simulink model "dynamik_6DoF"  (R2025b)
settings: Solver=VariableStepAuto  StartTime=0.0  StopTime=10.0  RelTol=1e-3
undefined symbols (not defined in the file): g, h0, Ivec, m
settings Model: Creator=chris  LastModifiedBy=chris
settings ModelReferenceCC: ModelReferenceMinAlgLoopOccurrences=on

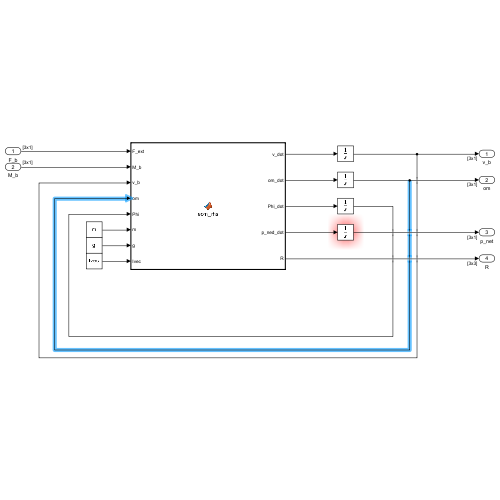
[thumbnail: Simulink's stored preview of the top-level diagram]
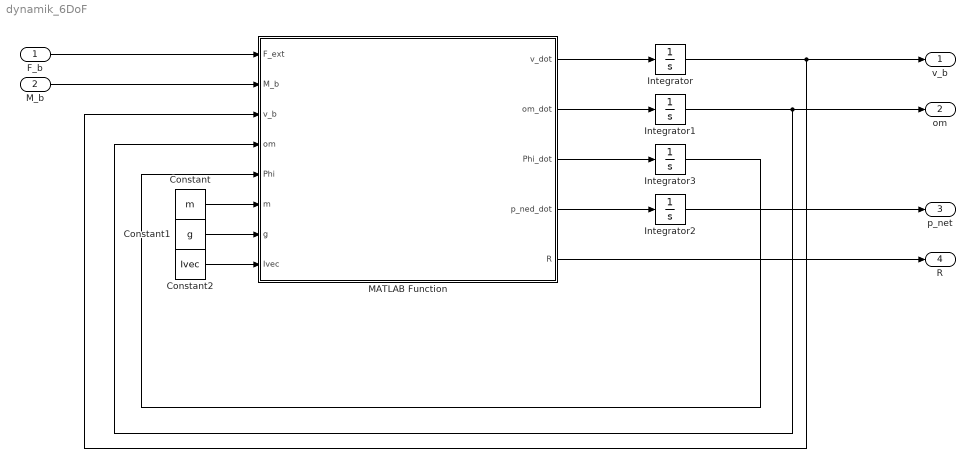
== system dynamik_6DoF ==
  F_b : Inport  PortDimensions=[3 1]
  M_b : Inport  Port=2  PortDimensions=[3 1]
  Constant : Constant  Value=m
  Constant1 : Constant  Value=g
  Constant2 : Constant  Value=Ivec
  Integrator : Integrator  InitialCondition=[0;0;0]
  Integrator1 : Integrator  InitialCondition=[0;0;0]
  Integrator2 : Integrator  InitialCondition=[0;0;-h0]
  Integrator3 : Integrator  InitialCondition=[0;0;0]
  MATLAB Function : MATLAB Function  TreatAsAtomicUnit=on
  v_b : Outport  PortDimensions=[3 1]
  om : Outport  Port=2  PortDimensions=[3 1]
  p_net : Outport  Port=3  PortDimensions=[3 1]
  R : Outport  Port=4  PortDimensions=[3 3]
  wires:
  F_b/1 -> MATLAB Function/1(F_ext)
  M_b/1 -> MATLAB Function/2(M_b)
  MATLAB Function/1(v_dot) -> Integrator/1
  MATLAB Function/2(om_dot) -> Integrator1/1
  MATLAB Function/4(p_ned_dot) -> Integrator2/1
  MATLAB Function/3(Phi_dot) -> Integrator3/1
  Integrator/1 -> v_b/1, MATLAB Function/3(v_b)
  Integrator1/1 -> om/1, MATLAB Function/4(om)
  Integrator3/1 -> MATLAB Function/5(Phi)
  Constant/1 -> MATLAB Function/6(m)
  Constant1/1 -> MATLAB Function/7(g)
  Constant2/1 -> MATLAB Function/8(Ivec)
  MATLAB Function/5(R) -> R/1
  Integrator2/1 -> p_net/1

== matlab function dynamik_6DoF/MATLAB Function ==
  data: F_ext input; v_dot output; M_b input; v_b input; om input; Phi input; m input; g input; Ivec input; om_dot output; Phi_dot output size=[3 1]; p_ned_dot output; R output
function [v_dot, om_dot, Phi_dot, p_ned_dot, R] = eom_rhs(F_ext, M_b, v_b, om, Phi, m, g, Ivec)
% Rechte Seite aller 12 DGL. F_ext = Schub + Drag (Body), OHNE Gravitation.
phi = Phi(1); the = Phi(2); psi = Phi(3);
cph=cos(phi); sph=sin(phi); cth=cos(the); sth=sin(the); cps=cos(psi); sps=sin(psi);

% Rotationsmatrix Body->NED (ZYX), Gl. (4.5)
R = [cth*cps, sph*sth*cps-cph*sps, cph*sth*cps+sph*sps;
     cth*sps, sph*sth*sps+cph*cps, cph*sth*sps-sph*cps;
    -sth,     sph*cth,             cph*cth];

% Gravitation in den Body-Frame drehen (R' = NED->Body)
F_grav_b = R.' * [0; 0; m*g];

v_dot     = (F_ext + F_grav_b)/m - cross(om, v_b);   % (4.1)
om_dot    = (M_b - cross(om, Ivec.*om)) ./ Ivec;     % (4.2)
W = [1, sph*tan(the), cph*tan(the);                  % (4.3) Sing. bei the=±pi/2
     0, cph,         -sph;
     0, sph/cth,      cph/cth];
Phi_dot   = W * om;
p_ned_dot = R * v_b;                                 % (4.4)
end
